simulink model "PIDControl"  (R2022a)
settings: Solver=VariableStepAuto  StartTime=0.0  StopTime=30  MaxStep=0.0001  RelTol=1e-3
undefined symbols (not defined in the file): q01, q02, tau0
libraries: slpidlib x2
settings Model: Creator=y.briere  LastModifiedBy=fades
settings DebuggingCC: UnconnectedInputMsg=warning  UnconnectedOutputMsg=warning  UnconnectedLineMsg=warning
settings RTWCC: DLArmComputeVersion=19.05

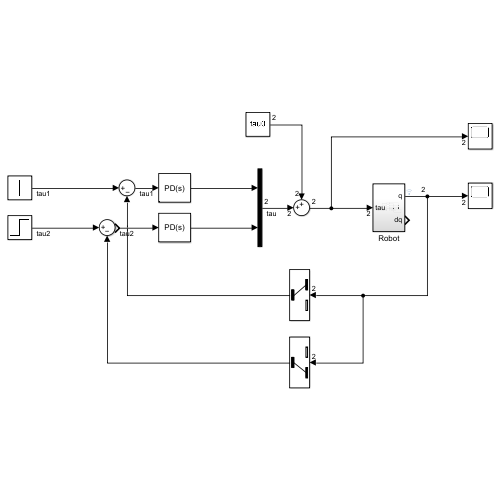
[thumbnail: Simulink's stored preview of the top-level diagram]
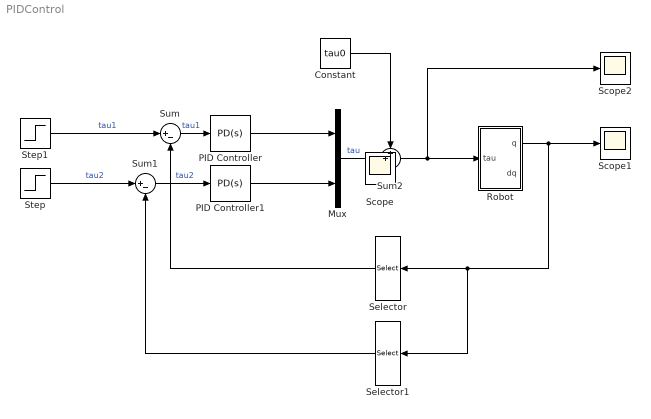
== system PIDControl ==
  Constant : Constant  Value=tau0
  Mux : Mux  Inputs=2
  PID Controller : slpidlib/PID Controller  Controller=PD  Form=Parallel  TimeDomain=Continuous-time  UseExternalTs=off  SampleTime=-1  IntegratorMethod=Forward Euler  FilterMethod=Forward Euler  ControllerParametersSource=internal  P=2.81971026283702  I=29.4445784073949  UseKiTs=off  D=3.33580713123512  N=169.76403442381  UseFilter=on  TunerSelectOption=Transfer Function Based (PID Tuner App)  InitialConditionSource=internal  InitialConditionForIntegrator=0  InitialConditionForFilter=0  DifferentiatorICPrevScaledInput=0  ExternalReset=none  TrackingMode=off  Kt=1  LimitOutput=off  SatLimitsSource=internal  UpperSaturationLimit=inf  LowerSaturationLimit=-inf  LinearizeAsGain=on  AntiWindupMode=none  Kb=1  POutMin=[]  POutMax=[]  IOutMin=[]  IOutMax=[]  DOutMin=[]  DOutMax=[]  NOutMin=[]  NOutMax=[]  SumOutMin=[]  SumOutMax=[]  SaturationOutMin=[]  SaturationOutMax=[]  PParamMin=[]  PParamMax=[]  IParamMin=[]  IParamMax=[]  DParamMin=[]  DParamMax=[]  NParamMin=[]  NParamMax=[]  KbParamMin=[]  KbParamMax=[]  KtParamMin=[]  KtParamMax=[]  KbOutMin=[]  KbOutMax=[]  KtOutMin=[]  KtOutMax=[]  IntegratorOutMin=[]  IntegratorOutMax=[]  FilterOutMin=[]  FilterOutMax=[]  SumI1OutMin=[]  SumI1OutMax=[]  SumI2OutMin=[]  SumI2OutMax=[]  SumI3OutMin=[]  SumI3OutMax=[]  SumI4OutMin=[]  SumI4OutMax=[]  SumDOutMin=[]  SumDOutMax=[]  DifferentiatorOutMin=[]  DifferentiatorOutMax=[]  FilterDiffOutCoefMin=[]  FilterDiffOutCoefMax=[]  ReciprocalOutMin=[]  ReciprocalOutMax=[]  SumDenOutMin=[]  SumDenOutMax=[]  SumNumOutMin=[]  SumNumOutMax=[]  DivideOutMin=[]  DivideOutMax=[]  UdiffTsProdOutMin=[]  UdiffTsProdOutMax=[]  NTsProdOutMin=[]  NTsProdOutMax=[]  UintegralTsProdOutMin=[]  UintegralTsProdOutMax=[]  UngainTsProdOutMin=[]  UngainTsProdOutMax=[]  IntegratorContinuousStateAttributes=''  IntegratorStateMustResolveToSignalObject=off  IntegratorRTWStateStorageClass=Auto  FilterContinuousStateAttributes=''  FilterStateMustResolveToSignalObject=off  FilterRTWStateStorageClass=Auto  ParallelPVariant=InternalParameters  IdealPVariant=Disabled  IVariant=Disabled  DVariant=InternalParameters  IntegratorVariant=Disabled  SatVariant=Disabled  AWVariant=Disabled  PCopyVariant=Disabled  TRVariant=Disabled  FdbkBlocksVariant=Forward  IdealPFdbkVariant=Disabled  SatFdbkVariant=Disabled  DerivativeFilterVariant=ContFilter  NVariant=InternalParameters  NCopyVariant=Disabled  FilterICVariant=InternalICsFilter  IntegratorICVariant=Disabled  ExternalResetVariant=Disabled  TRSumVariant=Passthrough  SumFdbkVariant=Disabled  SumVariant=Sum_PD  TsampFilterVariant=InternalTs  TsampNgainVariant=Passthrough  TsampIntegralVariant=Disabled_SignalSpec  ExternalSaturationOutDataTypeStr=Inherit: Same as second input  aMode=0
  PID Controller1 : slpidlib/PID Controller  Controller=PD  Form=Parallel  TimeDomain=Continuous-time  UseExternalTs=off  SampleTime=-1  IntegratorMethod=Forward Euler  FilterMethod=Forward Euler  ControllerParametersSource=internal  P=71.8655656673028  I=2.77895592487954  UseKiTs=off  D=0.701552085992472  N=114.441786456132  UseFilter=on  TunerSelectOption=Transfer Function Based (PID Tuner App)  InitialConditionSource=internal  InitialConditionForIntegrator=0  InitialConditionForFilter=0  DifferentiatorICPrevScaledInput=0  ExternalReset=none  TrackingMode=off  Kt=1  LimitOutput=off  SatLimitsSource=internal  UpperSaturationLimit=inf  LowerSaturationLimit=-inf  LinearizeAsGain=on  AntiWindupMode=none  Kb=1  POutMin=[]  POutMax=[]  IOutMin=[]  IOutMax=[]  DOutMin=[]  DOutMax=[]  NOutMin=[]  NOutMax=[]  SumOutMin=[]  SumOutMax=[]  SaturationOutMin=[]  SaturationOutMax=[]  PParamMin=[]  PParamMax=[]  IParamMin=[]  IParamMax=[]  DParamMin=[]  DParamMax=[]  NParamMin=[]  NParamMax=[]  KbParamMin=[]  KbParamMax=[]  KtParamMin=[]  KtParamMax=[]  KbOutMin=[]  KbOutMax=[]  KtOutMin=[]  KtOutMax=[]  IntegratorOutMin=[]  IntegratorOutMax=[]  FilterOutMin=[]  FilterOutMax=[]  SumI1OutMin=[]  SumI1OutMax=[]  SumI2OutMin=[]  SumI2OutMax=[]  SumI3OutMin=[]  SumI3OutMax=[]  SumI4OutMin=[]  SumI4OutMax=[]  SumDOutMin=[]  SumDOutMax=[]  DifferentiatorOutMin=[]  DifferentiatorOutMax=[]  FilterDiffOutCoefMin=[]  FilterDiffOutCoefMax=[]  ReciprocalOutMin=[]  ReciprocalOutMax=[]  SumDenOutMin=[]  SumDenOutMax=[]  SumNumOutMin=[]  SumNumOutMax=[]  DivideOutMin=[]  DivideOutMax=[]  UdiffTsProdOutMin=[]  UdiffTsProdOutMax=[]  NTsProdOutMin=[]  NTsProdOutMax=[]  UintegralTsProdOutMin=[]  UintegralTsProdOutMax=[]  UngainTsProdOutMin=[]  UngainTsProdOutMax=[]  IntegratorContinuousStateAttributes=''  IntegratorStateMustResolveToSignalObject=off  IntegratorRTWStateStorageClass=Auto  FilterContinuousStateAttributes=''  FilterStateMustResolveToSignalObject=off  FilterRTWStateStorageClass=Auto  ParallelPVariant=InternalParameters  IdealPVariant=Disabled  IVariant=Disabled  DVariant=InternalParameters  IntegratorVariant=Disabled  SatVariant=Disabled  AWVariant=Disabled  PCopyVariant=Disabled  TRVariant=Disabled  FdbkBlocksVariant=Forward  IdealPFdbkVariant=Disabled  SatFdbkVariant=Disabled  DerivativeFilterVariant=ContFilter  NVariant=InternalParameters  NCopyVariant=Disabled  FilterICVariant=InternalICsFilter  IntegratorICVariant=Disabled  ExternalResetVariant=Disabled  TRSumVariant=Passthrough  SumFdbkVariant=Disabled  SumVariant=Sum_PD  TsampFilterVariant=InternalTs  TsampNgainVariant=Passthrough  TsampIntegralVariant=Disabled_SignalSpec  ExternalSaturationOutDataTypeStr=Inherit: Same as second input  aMode=0
  Robot : Subsystem
  Scope1 : Scope
  Scope2 : Scope
  Selector : Selector  InputPortWidth=2  IndexOptions=Index vector (dialog)  Indices=1  OutputSizes=1
  Selector1 : Selector  InputPortWidth=2  IndexOptions=Index vector (dialog)  Indices=2  OutputSizes=1
  Step : Step  Before=q02  After=q02  SampleTime=0
  Step1 : Step  Before=q01  After=q01+0.5  SampleTime=0
  Sum : Sum  Inputs=|+-
  Sum1 : Sum  Inputs=|+-
  Sum2 : Sum  Inputs=++|
  Scope : Scope
  wires:
  Sum1/1 -> PID Controller1/1  "tau2"
  Sum/1 -> PID Controller/1  "tau1"
  Step1/1 -> Sum/1  "tau1"
  Step/1 -> Sum1/1  "tau2"
  Selector/1 -> Sum/2
  Selector1/1 -> Sum1/2
  Robot/1(q) -> Selector1/1, Selector/1, Scope1/1
  PID Controller/1 -> Mux/1
  PID Controller1/1 -> Mux/2
  Mux/1 -> Sum2/2  "tau"
  Sum2/1 -> Scope2/1, Robot/1(tau)
  Constant/1 -> Sum2/1

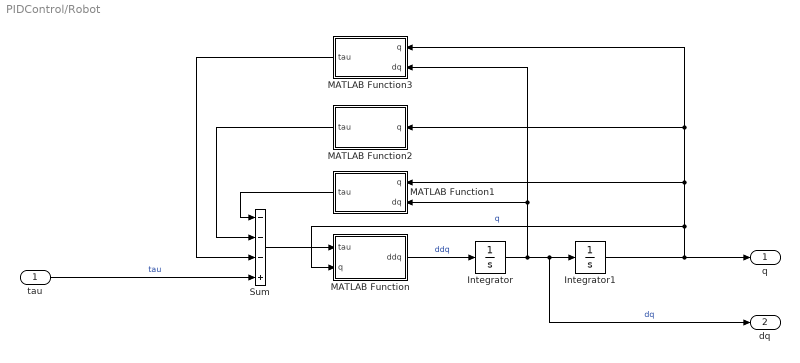
== system PIDControl/Robot ==
  tau : Inport
  Integrator : Integrator  InitialCondition=[0:0]
  Integrator1 : Integrator  InitialCondition=[q01;q02]
  MATLAB Function : MATLAB Function  TreatAsAtomicUnit=on
  MATLAB Function1 : MATLAB Function  TreatAsAtomicUnit=on
  MATLAB Function2 : MATLAB Function  TreatAsAtomicUnit=on
  MATLAB Function3 : MATLAB Function  TreatAsAtomicUnit=on
  Sum : Sum  Inputs=---+
  q : Outport
  dq : Outport  Port=2
  wires:
  Integrator/1 -> MATLAB Function3/2(dq), MATLAB Function1/2(dq), dq/1, Integrator1/1  "dq"
  Integrator1/1 -> MATLAB Function3/1(q), MATLAB Function2/1(q), MATLAB Function1/1(q), MATLAB Function/2(q), q/1  "q"
  MATLAB Function3/1(tau) -> Sum/3
  MATLAB Function/1(ddq) -> Integrator/1  "ddq"
  Sum/1 -> MATLAB Function/1(tau)
  MATLAB Function1/1(tau) -> Sum/1
  MATLAB Function2/1(tau) -> Sum/2
  tau/1 -> Sum/4  "tau"

== matlab function PIDControl/Robot/MATLAB Function1 ==
  data: q input; dq input; tau output
function tau  = coriolis(q,dq)
% Convective Matrix
%Robot parameters
R.m1 = 1; % Arm 1 mass
R.m2 = 1; % Arm 2 mass
R.L1 = 1; % Arm 1 length
R.L2 = 1; % Arm 2 length
Cm = [-R.m2*R.L1*R.L2*sin(q(2))*dq(2) -R.m2*R.L1*R.L2*sin(q(2))/2*dq(2);...
    R.m2*R.L1*R.L2*dq(1)*sin(q(2))/2 0];
tau = Cm*dq;

== matlab function PIDControl/Robot/MATLAB Function ==
  data: tau input; q input; ddq output
function ddq  = invM(tau,q)
% Mass matrix
R.m1 = 1; % Arm 1 mass
R.m2 = 1; % Arm 2 mass
R.L1 = 1; % Arm 1 length
R.L2 = 1; % Arm 2 length
M = [(R.m1*R.L1^2)/4+R.m2*(R.L1^2+R.L2^2/4+R.L1*R.L2*cos(q(2))) ,  R.m2*R.L2*(R.L2+ 2*R.L1*cos(q(2)))/4
    R.m2*R.L2*(R.L2+ 2*R.L1*cos(q(2)))/4                       ,  R.m2*R.L2^2/4];

ddq = M\tau;

== matlab function PIDControl/Robot/MATLAB Function2 ==
  data: q input; tau output
function tau  = gravity(q)
%Robot parameters
R.m1 = 1; % Arm 1 mass
R.m2 = 1; % Arm 2 mass
R.L1 = 1; % Arm 1 length
R.L2 = 1; % Arm 2 length
R.g = -0*9.81; % Gravity

tau = [R.m1*R.g*R.L1*cos(q(1))/2+R.m2*R.g*(R.L2*cos(q(1)+q(2))/2+R.L1*cos(q(1)));...
    R.m2*R.g*R.L2*cos(q(1)+q(2))/2];

== matlab function PIDControl/Robot/MATLAB Function3 ==
  data: q input; dq input; tau output
function tau  = friction(q,dq)
%Robot parameters
R.f1 = 1; % Friction 1
R.f2 = 1; % Friction 2

tau = [R.f1
    R.f2].*dq;
